simulink model "StateSpacev2"  (R2021b)
settings: Solver=FixedStepAuto  StartTime=0.0  StopTime=100  FixedStep=1e-3  RelTol=1e-3
values from neighbouring files (symbols this model uses):
  depth = -30 * 1e-3    (= -0.03)    [changing_acc.m]    (also in changing_depth.m; dostateSpacev2.m; forward_control.m)
  holdtime = 0.5    [dostateSpacev2.m]    (also in forward_control.m)
undefined symbols (not defined in the file or in its folder): vel
libraries: simulink x5
settings Model: Creator=HuijiangWang  LastModifiedBy=Emily

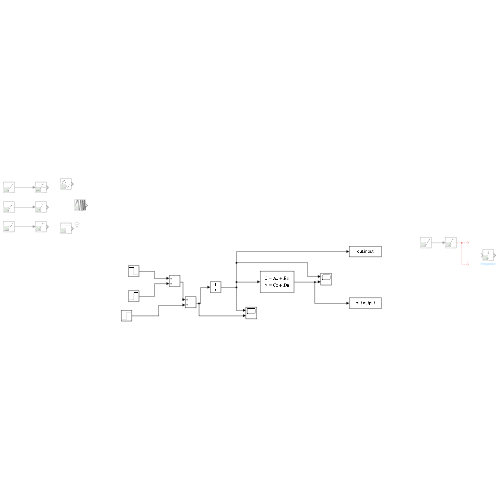
[thumbnail: Simulink's stored preview of the top-level diagram]
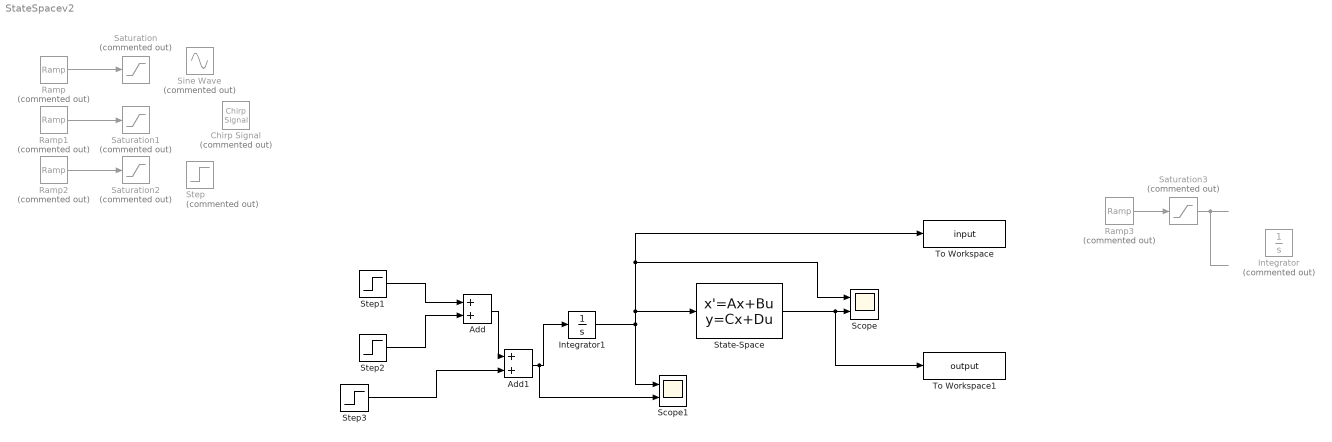
== system StateSpacev2 ==
  Add : Sum
  Add1 : Sum
  Chirp Signal : simulink/Sources/Chirp Signal  Commented=on  f1=0.1  T=100  f2=1
  Integrator : Integrator  Commented=on
  Integrator1 : Integrator
  Ramp : simulink/Sources/Ramp  Commented=on  slope=vel  start=0  InitialOutput=0
  Ramp1 : simulink/Sources/Ramp  Commented=on  slope=0.5  start=0  InitialOutput=0
  Ramp2 : simulink/Sources/Ramp  Commented=on  slope=0.2  start=0  InitialOutput=0
  Ramp3 : simulink/Sources/Ramp  Commented=on  slope=-vel  start=0  InitialOutput=-vel
  Saturation : Saturate  Commented=on  UpperLimit=10  LowerLimit=depth
  Saturation1 : Saturate  Commented=on  UpperLimit=10  LowerLimit=-10
  Saturation2 : Saturate  Commented=on  UpperLimit=10  LowerLimit=-10
  Saturation3 : Saturate  Commented=on  UpperLimit=vel  LowerLimit=-vel
  Scope : Scope  NumInputPorts=2
  Scope1 : Scope  NumInputPorts=2
  Sine Wave : Sin  Commented=on  SampleTime=0
  State-Space : StateSpace  A=|  B=|  C=[1 0 0 0; 0 0 1 0]  D=[0; 0]  InitialCondition=0
      A=|
      | [0 1 0 0; 
      |     -(k0+k1)/m1 -(c0+c1)/m1 k1/m1 c1/m1;
      |     0 0 0 1; 
      |     k1/m2 c1/m2 -1*(k1+k2)/m2 -1*(c1+c2)/m2]
      B=|
      | [c0/m1;
      |     k0/m1-(c0^2+c0*c1)/m1^2;
      |     0;
      |     c0*c1/(m1*m2)]
  Step : Step  Commented=on  After=10  SampleTime=0
  Step1 : Step  Time=0  After=-vel  SampleTime=0
  Step2 : Step  Time=-depth/vel  After=vel  SampleTime=0
  Step3 : Step  Time=-depth/vel+holdtime  After=vel  SampleTime=0
  To Workspace : ToWorkspace  VariableName=input  SaveFormat=Timeseries  SampleTime=-1
  To Workspace1 : ToWorkspace  VariableName=output  SaveFormat=Timeseries  SampleTime=-1
  wires:
  Ramp/1 -> Saturation/1
  State-Space/1 -> To Workspace1/1, Scope/2
  Integrator1/1 -> Scope1/1, To Workspace/1, Scope/1, State-Space/1
  Ramp1/1 -> Saturation1/1
  Ramp2/1 -> Saturation2/1
  Saturation3/1 -> ?
  Ramp3/1 -> Saturation3/1
  Step1/1 -> Add/1
  Step2/1 -> Add/2
  Add/1 -> Add1/1
  Step3/1 -> Add1/2
  Add1/1 -> Scope1/2, Integrator1/1
